simulink model "sampleModel121"  (R2021b)
settings: Solver=VariableStepAuto  StartTime=0.0  StopTime=10.0  RelTol=1e-3
undefined symbols (not defined in the file or in its folder): DiscIntNeverNeededParam
libraries: simulink x5, slpidlib x1
settings Model: Creator=user  LastModifiedBy=user

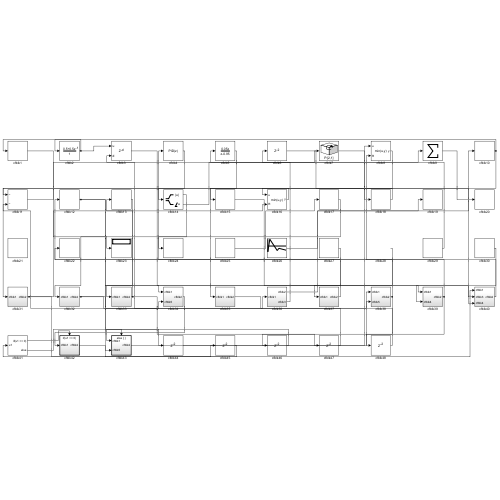
[thumbnail: Simulink's stored preview of the top-level diagram]
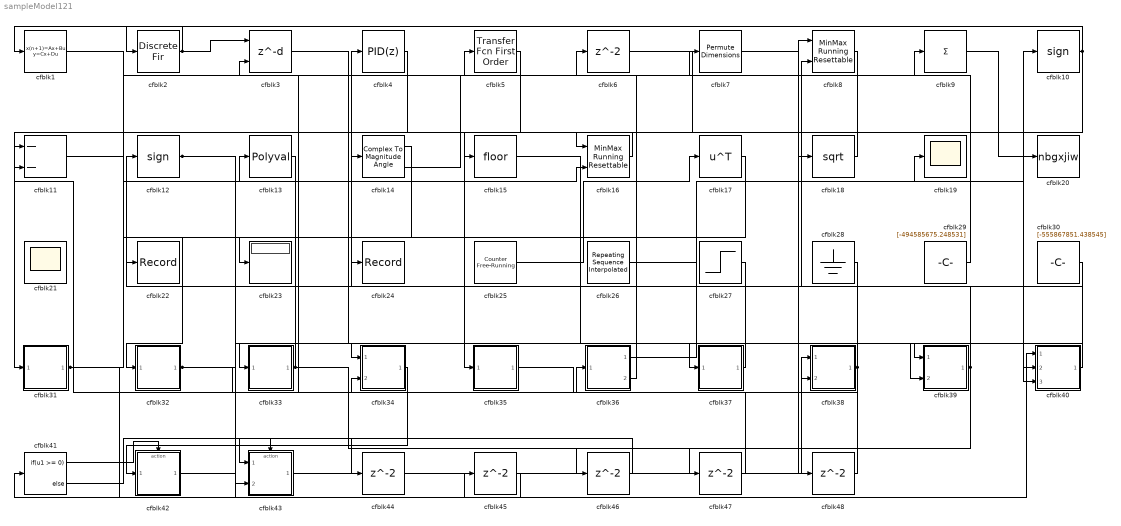
== system sampleModel121 ==
  cfblk1 : DiscreteStateSpace
  cfblk10 : Signum
  cfblk11 : Sum  Inputs=--
  cfblk12 : Signum
  cfblk13 : Polyval  Coefs=[ +2.081618890e-019, -1.441693666e-014, +4.719686976e-010, -8.536869453e-006, +1.621573104e-001, -8.087801117e+001 ]
  cfblk14 : ComplexToMagnitudeAngle
  cfblk15 : Rounding
  cfblk16 : simulink/Math Operations/MinMax Running Resettable  Function=min  vinit=0.0
  cfblk17 : Math  Operator=transpose  SaturateOnIntegerOverflow=on
  cfblk18 : Sqrt  SaturateOnIntegerOverflow=on
  cfblk19 : Scope
  cfblk2 : DiscreteFir  SampleTime=1
  cfblk20 : ToWorkspace  VariableName=nbgxjiw  SaveFormat=Timeseries  SampleTime=-1
  cfblk21 : Scope
      settings: Floating=on
  cfblk22 : Record  FileSettingsInternal="{\"entries\":[{\"content\":{\"excelSettings\":{\"content\":{},\"type\":\"Streamout.ExcelSettings\"}},\"type\":\"Streamout.FileSettingStorage\",\"uuid\":\"fd740401-2b8e-40f4-899f-90ca964aec60\"}],\"packageUris\":[\"http://schema.mathworks.com/mf0/streamout_blocks/R2020a\"],\"version\":\"1.0\"}"  SignalsInternal="{\"entries\":[{\"content\":{\"signals\":[{\"content\":{\"blockPath\":[\"sampleModel121/cfblk22\"],\"channel\":[],\"dimensions\":[1],\"domain\":\"sampleModel121/cfblk22\",\"lineColor\":\"#a2142f\",\"plots\":[1],\"port\":1,\"sid\":[\"\"],\"signalID\":4227,\"signalName\":\"cfblk33\"},\"type\":\"RecordBlkView.Signal\",\"uuid\":\"5daead5c-1d5e-454e-a752-94514f76c39d\"}]},\"type\":\"RecordBlkView.InputSignals\",\"uuid\":\"386915b9-b9f9-42da-b1ef-b10f4c0e1228\"}],\"packageUris\":[\"http://schema.mathworks.com/mf0/streamout_blocks/R2020a\"],\"version\":\"1.0\"}"  VisualizationBindings="{\"sparklinesplugin\":{\"info\":[{\"bindingParametersList\":[],\"subplotID\":1}]}}"
  cfblk23 : Display
  cfblk24 : Record  FileSettingsInternal="{\"entries\":[{\"content\":{\"excelSettings\":{\"content\":{},\"type\":\"Streamout.ExcelSettings\"}},\"type\":\"Streamout.FileSettingStorage\",\"uuid\":\"1580d6fb-15e4-47d5-8716-256e97cdfb47\"}],\"packageUris\":[\"http://schema.mathworks.com/mf0/streamout_blocks/R2020a\"],\"version\":\"1.0\"}"  SignalsInternal="{\"entries\":[{\"content\":{\"signals\":[{\"content\":{\"blockPath\":[\"sampleModel121/cfblk24\"],\"channel\":[],\"dimensions\":[1],\"domain\":\"sampleModel121/cfblk24\",\"lineColor\":\"#139fff\",\"plots\":[1],\"port\":1,\"sid\":[\"\"],\"signalID\":4231,\"signalName\":\"cfblk14:1\"},\"type\":\"RecordBlkView.Signal\",\"uuid\":\"eec9c35d-0f74-409a-8959-3dd03e3b2eaf\"}]},\"type\":\"RecordBlkView.InputSignals\",\"uuid\":\"52b8c401-7b59-45f7-a67f-61b4681157ad\"}],\"packageUris\":[\"http://schema.mathworks.com/mf0/streamout_blocks/R2020a\"],\"version\":\"1.0\"}"  VisualizationBindings="{\"sparklinesplugin\":{\"info\":[{\"bindingParametersList\":[],\"subplotID\":1}]}}"
  cfblk25 : simulink/Sources/Counter Free-Running  NumBits=[32.000000]  tsamp=-1
  cfblk26 : simulink/Sources/Repeating Sequence Interpolated  OutValues=[-846322446.587652, 994599961.907238, -684277103.208770, -321206679.696248, -632866226.506003]  TimeValues=[0 0.1 0.5 0.6 1].'  LookUpMeth=Use Input Above  tsamp=0.01  OutMin=[]  OutMax=[]  OutDataTypeStr=double  OutputDataTypeScalingMode=double  OutDataType=fixdt(0,8)  OutScaling=2^-10
  cfblk27 : Step  Time=[46.000000]  Before=[870636847.676478]  After=[-189163738.160871]  SampleTime=0
  cfblk28 : Ground
  cfblk29 : Constant  Value=[-494585675.248531]  SampleTime=1
  cfblk3 : Delay  DelayLengthSource=Input port  SampleTime=1
      settings: InputPortMap=u0,p1
  cfblk30 : Constant  Value=[-555867851.438545]  SampleTime=1
  cfblk31 : Subsystem
  cfblk32 : Subsystem
  cfblk33 : Subsystem
  cfblk34 : Subsystem
  cfblk35 : Subsystem
  cfblk36 : Subsystem
  cfblk37 : Subsystem
  cfblk38 : Subsystem
  cfblk39 : Subsystem
  cfblk4 : slpidlib/PID Controller  Controller=PID  Form=Parallel  TimeDomain=Discrete-time  UseExternalTs=off  SampleTime=1  IntegratorMethod=Forward Euler  FilterMethod=Forward Euler  ControllerParametersSource=internal  P=1  I=1  D=0  UseFilter=on  N=100  TunerSelectOption=Transfer Function Based (PID Tuner App)  InitialConditionSource=internal  InitialConditionForIntegrator=0  InitialConditionForFilter=0  DifferentiatorICPrevScaledInput=0  ExternalReset=none  TrackingMode=off  Kt=1  LimitOutput=off  SatLimitsSource=internal  UpperSaturationLimit=inf  LowerSaturationLimit=-inf  LinearizeAsGain=off  AntiWindupMode=none  Kb=1  POutMin=[]  POutMax=[]  IOutMin=[]  IOutMax=[]  DOutMin=[]  DOutMax=[]  NOutMin=[]  NOutMax=[]  SumOutMin=[]  SumOutMax=[]  SaturationOutMin=[]  SaturationOutMax=[]  PParamMin=[]  PParamMax=[]  IParamMin=[]  IParamMax=[]  DParamMin=[]  DParamMax=[]  NParamMin=[]  NParamMax=[]  KbParamMin=[]  KbParamMax=[]  KtParamMin=[]  KtParamMax=[]  KbOutMin=[]  KbOutMax=[]  KtOutMin=[]  KtOutMax=[]  IntegratorOutMin=[]  IntegratorOutMax=[]  FilterOutMin=[]  FilterOutMax=[]  SumI1OutMin=[]  SumI1OutMax=[]  SumI2OutMin=[]  SumI2OutMax=[]  SumI3OutMin=[]  SumI3OutMax=[]  SumI4OutMin=[]  SumI4OutMax=[]  SumDOutMin=[]  SumDOutMax=[]  DifferentiatorOutMin=[]  DifferentiatorOutMax=[]  FilterDiffOutCoefMin=[]  FilterDiffOutCoefMax=[]  ReciprocalOutMin=[]  ReciprocalOutMax=[]  SumDenOutMin=[]  SumDenOutMax=[]  SumNumOutMin=[]  SumNumOutMax=[]  DivideOutMin=[]  DivideOutMax=[]  UdiffTsProdOutMin=[]  UdiffTsProdOutMax=[]  NTsProdOutMin=[]  NTsProdOutMax=[]  UintegralTsProdOutMin=[]  UintegralTsProdOutMax=[]  UngainTsProdOutMin=[]  UngainTsProdOutMax=[]  IntegratorContinuousStateAttributes=''  IntegratorStateMustResolveToSignalObject=off  IntegratorRTWStateStorageClass=Auto  FilterContinuousStateAttributes=''  FilterStateMustResolveToSignalObject=off  FilterRTWStateStorageClass=Auto  ParallelPVariant=InternalParameters  IdealPVariant=Disabled  IVariant=InternalParameters  DVariant=InternalParameters  IntegratorVariant=Discrete  SatVariant=Disabled  AWVariant=Passthrough  PCopyVariant=Disabled  TRVariant=Disabled  FdbkBlocksVariant=Forward  IdealPFdbkVariant=Disabled  SatFdbkVariant=Disabled  DerivativeFilterVariant=ForwardEulerFilter  NVariant=InternalParameters  NCopyVariant=Disabled  FilterICVariant=InternalICsFilter  IntegratorICVariant=InternalICs  ExternalResetVariant=Disabled  TRSumVariant=Passthrough  SumFdbkVariant=Disabled  SumVariant=Sum_PID  TsampFilterVariant=InternalTs  TsampNgainVariant=Passthrough  TsampIntegralVariant=Passthrough  ExternalSaturationOutDataTypeStr=Inherit: Same as second input
  cfblk40 : Subsystem
  cfblk41 : If  IfExpression=u1 >= 0  SampleTime=1
  cfblk42 : Subsystem  TreatAsAtomicUnit=on
  cfblk43 : Subsystem  TreatAsAtomicUnit=on
  cfblk{6,44..48} (6 alike) : Delay  SampleTime=1
  cfblk5 : simulink/Discrete/Transfer Fcn First Order  PoleZ=0.95  ICPrevOutput=0.0  DoSatur=off
  cfblk7 : PermuteDimensions
  cfblk8 : simulink/Math Operations/MinMax Running Resettable  Function=min  vinit=0.0
  cfblk9 : Sum  Inputs=+
  wires:
  cfblk40/1(cfblk2) -> cfblk12/1
  cfblk18/1 -> cfblk31/1(cfblk1)
  cfblk29/1 -> cfblk5/1
  cfblk37/1(cfblk2) -> cfblk4/1
  cfblk33/1(cfblk2) -> cfblk22/1, cfblk47/1
  cfblk5/1 -> cfblk35/1(cfblk1)
  cfblk17/1 -> cfblk32/1(cfblk1)
  cfblk10/1 -> cfblk2/1, cfblk16/1
  cfblk9/1 -> cfblk20/1
  cfblk25/1 -> cfblk17/1
  cfblk13/1 -> cfblk33/1(cfblk1)
  cfblk16/1 -> cfblk15/1
  cfblk43/1(cfblk2) -> cfblk38/1(cfblk1)
  cfblk32/1(cfblk2) -> cfblk36/1(cfblk1), cfblk34/2(cfblk5)
  cfblk3/1 -> cfblk39/1(cfblk1)
  cfblk31/1(cfblk2) -> cfblk40/1(cfblk1), cfblk16/2
  cfblk38/1(cfblk2) -> cfblk13/1, cfblk46/1
  cfblk8/1 -> cfblk11/1
  cfblk15/1 -> cfblk40/2(cfblk3)
  cfblk35/1(cfblk2) -> cfblk38/2(cfblk5)
  cfblk36/1(cfblk2) -> cfblk19/1
  cfblk36/2(cfblk3) -> cfblk6/1
  cfblk12/1 -> cfblk34/1(cfblk1), cfblk44/1
  cfblk27/1 -> cfblk43/2(cfblk5)
  cfblk39/1(cfblk2) -> cfblk8/2, cfblk48/1
  cfblk7/1 -> cfblk18/1
  cfblk14/1 -> cfblk24/1
  cfblk28/1 -> cfblk37/1(cfblk1)
  cfblk1/1 -> cfblk23/1
  cfblk4/1 -> cfblk14/1
  cfblk14/2 -> cfblk9/1
  cfblk2/1 -> cfblk1/1, cfblk3/1
  cfblk34/1(cfblk2) -> cfblk42/1(cfblk1)
  cfblk30/1 -> cfblk39/2(cfblk4)
  cfblk26/1 -> cfblk10/1
  cfblk6/1 -> cfblk40/3(cfblk4)
  cfblk11/1 -> cfblk7/1
  cfblk41/1 -> cfblk42/Action
  cfblk41/2 -> cfblk43/Action
  cfblk44/1 -> cfblk8/1
  cfblk42/1(cfblk2) -> cfblk45/1
  cfblk45/1 -> cfblk41/1
  cfblk46/1 -> cfblk43/1(cfblk1)
  cfblk47/1 -> cfblk11/2
  cfblk48/1 -> cfblk3/2

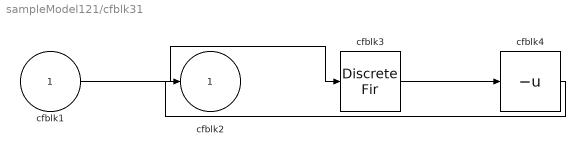
== system sampleModel121/cfblk31 ==
  cfblk1 : Inport
  cfblk3 : DiscreteFir  SampleTime=1
  cfblk4 : UnaryMinus
  cfblk2 : Outport
  wires:
  cfblk1/1 -> cfblk3/1
  cfblk3/1 -> cfblk4/1
  cfblk4/1 -> cfblk2/1

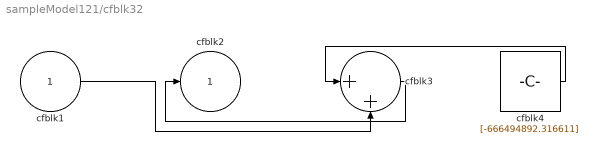
== system sampleModel121/cfblk32 ==
  cfblk1 : Inport
  cfblk3 : Sum  Inputs=|++
  cfblk4 : Constant  Value=[-666494892.316611]  SampleTime=1
  cfblk2 : Outport
  wires:
  cfblk4/1 -> cfblk3/1
  cfblk3/1 -> cfblk2/1
  cfblk1/1 -> cfblk3/2

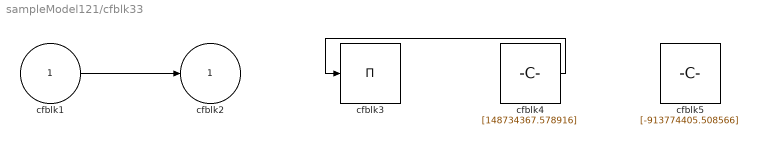
== system sampleModel121/cfblk33 ==
  cfblk1 : Inport
  cfblk3 : Product  Inputs=*
  cfblk4 : Constant  Value=[148734367.578916]  SampleTime=1
  cfblk5 : Constant  Value=[-913774405.508566]  SampleTime=1
  cfblk2 : Outport
  wires:
  cfblk4/1 -> cfblk3/1
  cfblk1/1 -> cfblk2/1

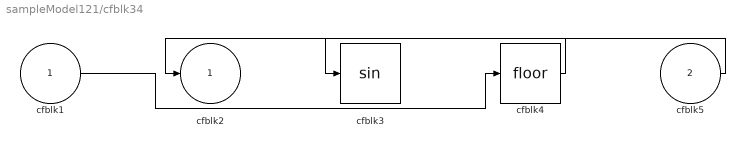
== system sampleModel121/cfblk34 ==
  cfblk1 : Inport
  cfblk5 : Inport  Port=2
  cfblk3 : Trigonometry
  cfblk4 : Rounding
  cfblk2 : Outport
  wires:
  cfblk4/1 -> cfblk2/1
  cfblk1/1 -> cfblk4/1
  cfblk5/1 -> cfblk3/1

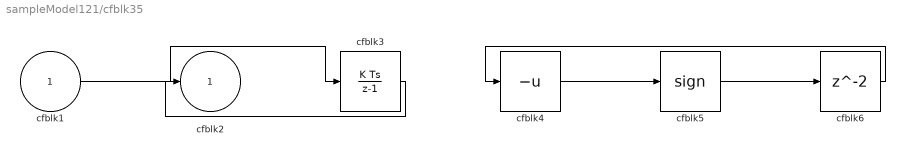
== system sampleModel121/cfblk35 ==
  cfblk1 : Inport
  cfblk3 : DiscreteIntegrator  ICPrevOutput=DiscIntNeverNeededParam  ICPrevScaledInput=DiscIntNeverNeededParam
  cfblk4 : UnaryMinus
  cfblk5 : Signum
  cfblk6 : Delay  SampleTime=1
  cfblk2 : Outport
  wires:
  cfblk4/1 -> cfblk5/1
  cfblk1/1 -> cfblk3/1
  cfblk3/1 -> cfblk2/1
  cfblk5/1 -> cfblk6/1
  cfblk6/1 -> cfblk4/1

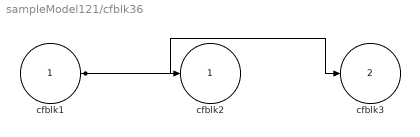
== system sampleModel121/cfblk36 ==
  cfblk1 : Inport
  cfblk2 : Outport
  cfblk3 : Outport  Port=2
  wires:
  cfblk1/1 -> cfblk3/1, cfblk2/1

== system sampleModel121/cfblk37 ==
  cfblk1 : Inport
  cfblk3 : Constant  Value=[-743175022.866624]  SampleTime=1
  cfblk2 : Outport
  wires:
  cfblk3/1 -> cfblk2/1

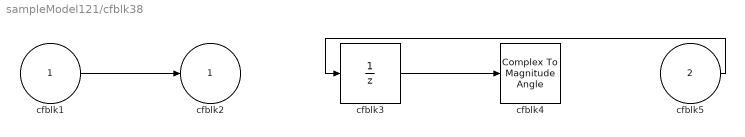
== system sampleModel121/cfblk38 ==
  cfblk1 : Inport
  cfblk5 : Inport  Port=2
  cfblk3 : UnitDelay  HasFrameUpgradeWarning=on
  cfblk4 : ComplexToMagnitudeAngle
  cfblk2 : Outport
  wires:
  cfblk1/1 -> cfblk2/1
  cfblk3/1 -> cfblk4/1
  cfblk5/1 -> cfblk3/1

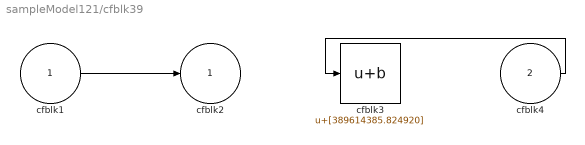
== system sampleModel121/cfblk39 ==
  cfblk1 : Inport
  cfblk4 : Inport  Port=2
  cfblk3 : Bias  Bias=[389614385.824920]
  cfblk2 : Outport
  wires:
  cfblk1/1 -> cfblk2/1
  cfblk4/1 -> cfblk3/1

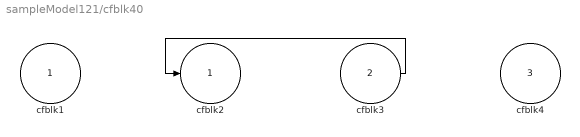
== system sampleModel121/cfblk40 ==
  cfblk1 : Inport
  cfblk3 : Inport  Port=2
  cfblk4 : Inport  Port=3
  cfblk2 : Outport
  wires:
  cfblk3/1 -> cfblk2/1

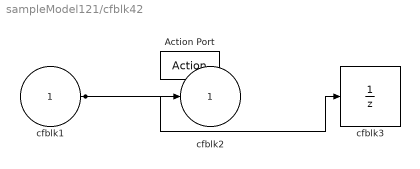
== system sampleModel121/cfblk42 ==
  cfblk1 : Inport
  Action Port : ActionPort  ActionPortLabel=if(u1 >= 0)
  cfblk3 : UnitDelay  SampleTime=-1  HasFrameUpgradeWarning=on
  cfblk2 : Outport
  wires:
  cfblk1/1 -> cfblk2/1, cfblk3/1

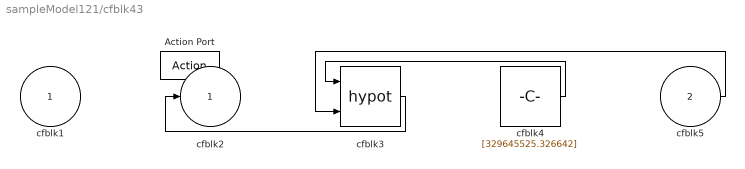
== system sampleModel121/cfblk43 ==
  cfblk1 : Inport
  cfblk5 : Inport  Port=2
  Action Port : ActionPort  ActionPortLabel=else
  cfblk3 : Math  Operator=hypot  SaturateOnIntegerOverflow=on
  cfblk4 : Constant  Value=[329645525.326642]  SampleTime=1
  cfblk2 : Outport
  wires:
  cfblk4/1 -> cfblk3/1
  cfblk3/1 -> cfblk2/1
  cfblk5/1 -> cfblk3/2
